simulink model "modelo_dp_mod_am"  (R2024b)
settings: Solver=VariableStepDiscrete  StartTime=0.0  StopTime=sim_time  RelTol=1e-3  EnableMultiTasking=on
values from neighbouring files (symbols this model uses):
  f_cic_scale = ceil(log2(G_cic_int))    [conf_mod_filter_design_p1_2.m]
  fc = 30    [configura_modelo_dp_mod_am.m]
  fmod = 20    [configura_modelo_dp_mod_am.m]
  fsc = 96    [configura_modelo_dp_mod_am.m]
  h_comp_cic = round(h_comp_cic*2^16)*2^-16    [conf_mod_filter_design_p1_2.m]
  h_comp_DAC = [-1/16 1-2^-3 -1/16]    [conf_mod_filter_design_p1_2.m]
  m_am = 1*(1-2^-15)    (= 0.999969482422)    [configura_modelo_dp_mod_am.m]
  R = 2000    [conf_mod_filter_design_p1_2.m]
undefined symbols (not defined in the file or in its folder): dspblkCoreblockFVToolHelper, gcbh
libraries: dspsigops x4, simulink x1, dspsrcs4 x1
settings Model: Creator=jvalls  LastModifiedBy=garto
settings SolverCC: AlgebraicLoopSolver=TrustRegion
settings DataIOCC: LimitDataPoints=on  SaveFormat=Array  ReturnWorkspaceOutputs=off
settings OptimizationCC: LifeSpan=inf
settings DebuggingCC: SolverPrmCheckMsg=warning  UnconnectedInputMsg=warning  UnconnectedOutputMsg=warning  UnconnectedLineMsg=warning  SFUnexpectedBacktrackingDiag=warning  SFNoUnconditionalDefaultTransitionDiag=warning  SFExecutionAtInitializationDiag=none  ArithmeticOperatorsInVariantConditions=warning
settings HardwareCC: ProdBitPerPointer=32  ProdBitPerSizeT=32  ProdBitPerPtrDiffT=32  ProdLargestAtomicFloat=None  ProdIntDivRoundTo=Undefined  ProdEndianess=Unspecified  ProdWordSize=32  ProdHWDeviceType=32-bit Generic
settings ModelReferenceCC: EnableRefExpFcnMdlSchedulingChecks=on  PropagateSignalLabelsOutOfModel=off
settings SFSimCC: SimUseLocalCustomCode=off  CustomCodeUndefinedFunction=UseInterfaceOnly
settings RTWCC: RTWUseLocalCustomCode=off  GPUComputeCapability=3.5
settings CodeAppCC: StateflowObjectComments=on
settings GRTTargetCC: TargetLangStandard=C89/C90 (ANSI)
settings ConfigComp: CovMetricSettings=dw  CovSaveCumulativeToWorkspaceVar=on  CovSaveSingleToWorkspaceVar=on  CovExternalEMLEnable=off  CovSFcnEnable=off

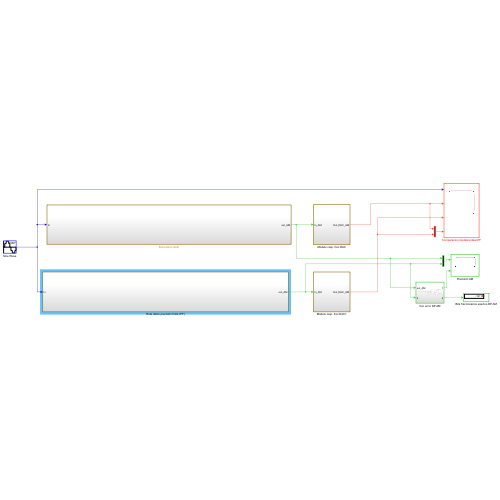
[thumbnail: Simulink's stored preview of the top-level diagram]
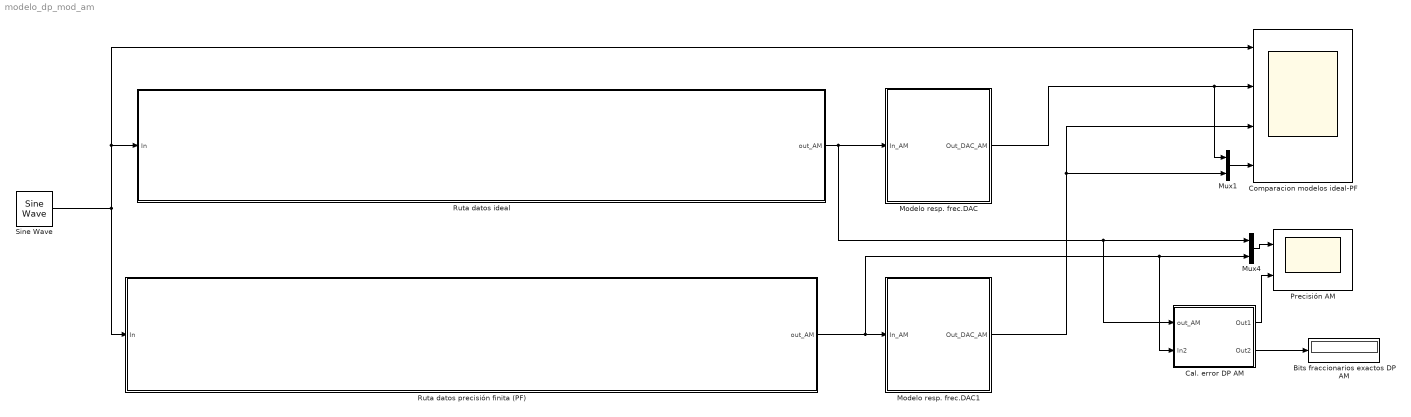
== system modelo_dp_mod_am ==
  Bits fraccionarios exactos DP AM : Display
  Cal. error DP AM : Subsystem
  Comparacion modelos ideal-PF : Scope  NumInputPorts=4
  Modelo resp. frec.DAC : Subsystem
  Modelo resp. frec.DAC1 : Subsystem
  Mux1 : Mux  Inputs=2
  Mux4 : Mux  Inputs=2
  Precisión AM : Scope  NumInputPorts=2
  Ruta datos ideal : Subsystem
  Ruta datos precisión finita (PF) : Subsystem
  Sine Wave : dspsrcs4/Sine Wave  Amplitude=1-2^-15  Frequency=fmod*1e-3  Phase=0  SampleMode=Discrete  OutComplex=Real  CompMethod=Trigonometric fcn  TableSize=Speed  SampleTime=R/fsc  SamplesPerFrame=1  ResetState=Restart at time zero  OutputFrames=off  dataType=double  wordLen=16  udDataType=sfix(16)  fracBitsMode=Best precision  numFracBits=15  OutDataTypeStr=double  LastOutDataTypeStr=double
  wires:
  Mux1/1 -> Comparacion modelos ideal-PF/4
  Modelo resp. frec.DAC/1(Out_DAC_AM) -> Mux1/1, Comparacion modelos ideal-PF/2
  Modelo resp. frec.DAC1/1(Out_DAC_AM) -> Comparacion modelos ideal-PF/3, Mux1/2
  Ruta datos ideal/1(out_AM) -> Cal. error DP AM/1(out_AM), Mux4/1, Modelo resp. frec.DAC/1(In_AM)
  Ruta datos precisión finita (PF)/1(out_AM) -> Cal. error DP AM/2(In2), Mux4/2, Modelo resp. frec.DAC1/1(In_AM)
  Cal. error DP AM/1(Out1) -> Precisión AM/2
  Cal. error DP AM/2(Out2) -> Bits fraccionarios exactos DP AM/1
  Sine Wave/1 -> Comparacion modelos ideal-PF/1, Ruta datos ideal/1(In), Ruta datos precisión finita (PF)/1(In)
  Mux4/1 -> Precisión AM/1

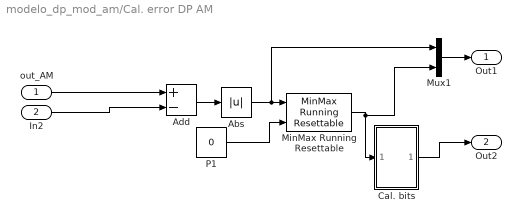
== system modelo_dp_mod_am/Cal. error DP AM ==
  out_AM : Inport
  In2 : Inport  Port=2
  Abs : Abs  SaturateOnIntegerOverflow=off
  Add : Sum  Inputs=+-
  Cal. bits : Subsystem
  MinMax Running Resettable : simulink/Math Operations/MinMax Running Resettable  Function=max  vinit=0.0
  Mux1 : Mux  Inputs=2
  P1 : Constant  Value=0  OutDataTypeStr=double  SampleTime=-1
  Out1 : Outport  VectorParamsAs1DForOutWhenUnconnected=off
  Out2 : Outport  Port=2  VectorParamsAs1DForOutWhenUnconnected=off
  wires:
  In2/1 -> Add/2
  Abs/1 -> Mux1/1, MinMax Running Resettable/1
  MinMax Running Resettable/1 -> Mux1/2, Cal. bits/1(In1)
  out_AM/1 -> Add/1
  P1/1 -> MinMax Running Resettable/2
  Add/1 -> Abs/1
  Cal. bits/1(Out1) -> Out2/1
  Mux1/1 -> Out1/1

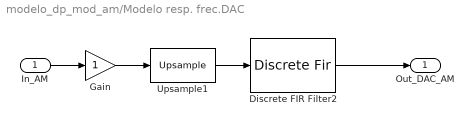
== system modelo_dp_mod_am/Modelo resp. frec.DAC ==
  In_AM : Inport
  Discrete FIR Filter2 : DiscreteFir  Coefficients=[1 1 1 1]  InputProcessing=Columns as channels (frame based)
  Gain : Gain  OutDataTypeStr=double
  Upsample1 : dspsigops/Upsample  FactorSource=Dialog parameter  N=4  Nmax=16  phase=0  InputProcessing=Columns as channels (frame based)  RateOptions=Allow multirate processing  ic=0  mode=Unused parameter value
  Out_DAC_AM : Outport  VectorParamsAs1DForOutWhenUnconnected=off
  wires:
  Upsample1/1 -> Discrete FIR Filter2/1
  Discrete FIR Filter2/1 -> Out_DAC_AM/1
  In_AM/1 -> Gain/1
  Gain/1 -> Upsample1/1

== system modelo_dp_mod_am/Modelo resp. frec.DAC1 ==
  In_AM : Inport
  Discrete FIR Filter2 : DiscreteFir  Coefficients=[1 1 1 1]  InputProcessing=Columns as channels (frame based)
  Gain : Gain  OutDataTypeStr=double
  Upsample1 : dspsigops/Upsample  FactorSource=Dialog parameter  N=4  Nmax=16  phase=0  InputProcessing=Columns as channels (frame based)  RateOptions=Allow multirate processing  ic=0  mode=Unused parameter value
  Out_DAC_AM : Outport  VectorParamsAs1DForOutWhenUnconnected=off
  wires:
  Upsample1/1 -> Discrete FIR Filter2/1
  Discrete FIR Filter2/1 -> Out_DAC_AM/1
  In_AM/1 -> Gain/1
  Gain/1 -> Upsample1/1

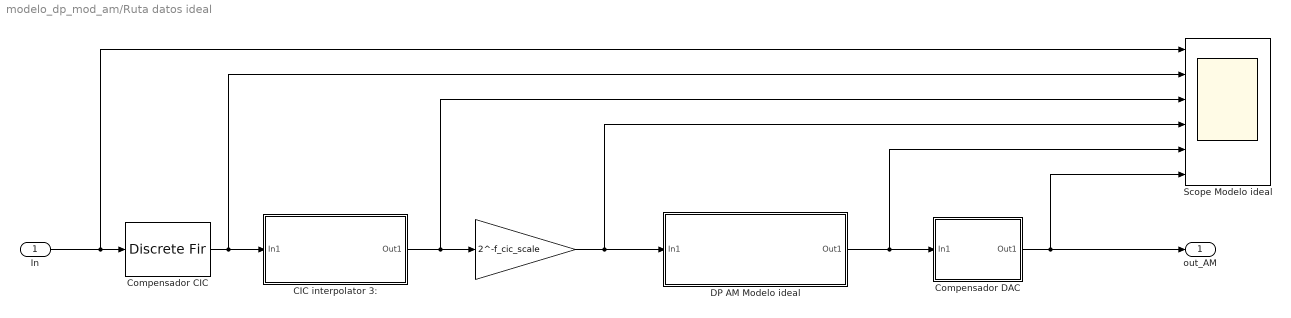
== system modelo_dp_mod_am/Ruta datos ideal ==
  In : Inport
  " " : Gain  Gain=2^-f_cic_scale  OutDataTypeStr=double
  "CIC interpolator 3: " : Subsystem
  Compensador CIC : DiscreteFir  LoadFcn=dspblkCoreblockFVToolHelper(gcbh,'load');  Coefficients=h_comp_cic  InputProcessing=Columns as channels (frame based)
      settings: CopyFcn=dspblkCoreblockFVToolHelper(gcbh,'copy');  DeleteFcn=dspblkCoreblockFVToolHelper(gcbh,'close');  ModelCloseFcn=dspblkCoreblockFVToolHelper(gcbh,'close');  PreSaveFcn=dspblkCoreblockFVToolHelper(gcbh,'presave');  PostSaveFcn=dspblkCoreblockFVToolHelper(gcbh,'postsave');  CloseFcn=dspblkCoreblockFVToolHelper(gcbh,'close');
  Compensador DAC : Subsystem
  DP AM Modelo ideal : Subsystem
  Scope Modelo ideal : Scope  NumInputPorts=6
  out_AM : Outport  VectorParamsAs1DForOutWhenUnconnected=off
  wires:
  "CIC interpolator 3: "/1(Out1) -> Scope Modelo ideal/3, " "/1
  " "/1 -> Scope Modelo ideal/4, DP AM Modelo ideal/1(In1)
  In/1 -> Scope Modelo ideal/1, Compensador CIC/1
  DP AM Modelo ideal/1(Out1) -> Compensador DAC/1(In1), Scope Modelo ideal/5
  Compensador CIC/1 -> Scope Modelo ideal/2, "CIC interpolator 3: "/1(In1)
  Compensador DAC/1(Out1) -> Scope Modelo ideal/6, out_AM/1

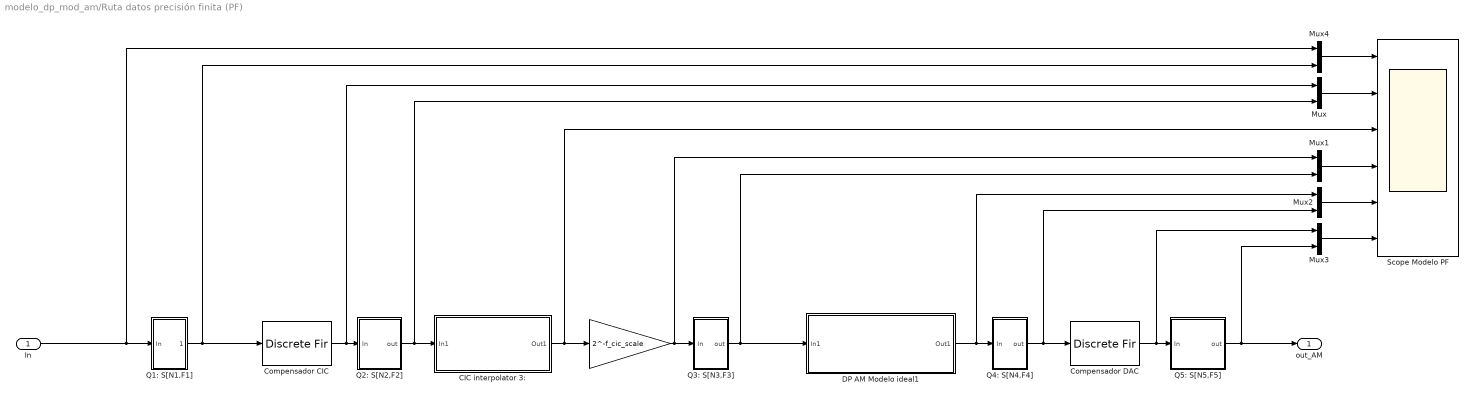
== system modelo_dp_mod_am/Ruta datos precisión finita (PF) ==
  In : Inport
  " " : Gain  Gain=2^-f_cic_scale  OutDataTypeStr=double
  "CIC interpolator 3: " : Subsystem
  Compensador CIC : DiscreteFir  LoadFcn=dspblkCoreblockFVToolHelper(gcbh,'load');  Coefficients=h_comp_cic  InputProcessing=Columns as channels (frame based)
      settings: CopyFcn=dspblkCoreblockFVToolHelper(gcbh,'copy');  DeleteFcn=dspblkCoreblockFVToolHelper(gcbh,'close');  ModelCloseFcn=dspblkCoreblockFVToolHelper(gcbh,'close');  PreSaveFcn=dspblkCoreblockFVToolHelper(gcbh,'presave');  PostSaveFcn=dspblkCoreblockFVToolHelper(gcbh,'postsave');  CloseFcn=dspblkCoreblockFVToolHelper(gcbh,'close');
  Compensador DAC : DiscreteFir  Coefficients=h_comp_DAC  InputProcessing=Columns as channels (frame based)
  DP AM Modelo ideal1 : Subsystem
  Mux{,1..4} (5 alike) : Mux  Inputs=2
  Q1: S[N1,F1] : Subsystem
  Q2: S[N2,F2] : Subsystem
  Q3: S[N3,F3] : Subsystem
  Q4: S[N4,F4] : Subsystem
  Q5: S[N5,F5] : Subsystem
  Scope Modelo PF : Scope  NumInputPorts=6
  out_AM : Outport  VectorParamsAs1DForOutWhenUnconnected=off
  wires:
  Compensador CIC/1 -> Mux/1, Q2: S[N2,F2]/1(In)
  " "/1 -> Q3: S[N3,F3]/1(In), Mux1/1
  DP AM Modelo ideal1/1(Out1) -> Mux2/1, Q4: S[N4,F4]/1(In)
  In/1 -> Mux4/1, Q1: S[N1,F1]/1(In)
  Q2: S[N2,F2]/1(out) -> Mux/2, "CIC interpolator 3: "/1(In1)
  Q3: S[N3,F3]/1(out) -> Mux1/2, DP AM Modelo ideal1/1(In1)
  Q5: S[N5,F5]/1(out) -> Mux3/2, out_AM/1
  "CIC interpolator 3: "/1(Out1) -> Scope Modelo PF/3, " "/1
  Q4: S[N4,F4]/1(out) -> Compensador DAC/1, Mux2/2
  Compensador DAC/1 -> Mux3/1, Q5: S[N5,F5]/1(In)
  Mux/1 -> Scope Modelo PF/2
  Mux1/1 -> Scope Modelo PF/4
  Mux2/1 -> Scope Modelo PF/5
  Mux3/1 -> Scope Modelo PF/6
  Q1: S[N1,F1]/1(Out1) -> Mux4/2, Compensador CIC/1
  Mux4/1 -> Scope Modelo PF/1

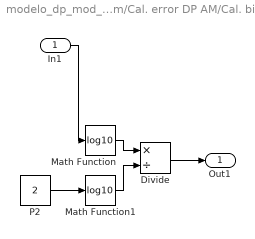
== system modelo_dp_mod_am/Cal. error DP AM/Cal. bits ==
  In1 : Inport
  Divide : Product  Inputs=*/
  Math Function : Math  Operator=log10  SignedPower=on
  Math Function1 : Math  Operator=log10  SignedPower=on
  P2 : Constant  Value=2  OutDataTypeStr=double  SampleTime=-1
  Out1 : Outport  VectorParamsAs1DForOutWhenUnconnected=off
  wires:
  P2/1 -> Math Function1/1
  Math Function1/1 -> Divide/2
  In1/1 -> Math Function/1
  Math Function/1 -> Divide/1
  Divide/1 -> Out1/1

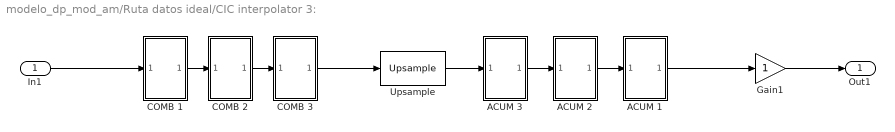
== system modelo_dp_mod_am/Ruta datos ideal/CIC interpolator 3:  ==
  In1 : Inport
  ACUM 1 : Subsystem
  ACUM 2 : Subsystem
  ACUM 3 : Subsystem
  COMB 1 : Subsystem
  COMB 2 : Subsystem
  COMB 3 : Subsystem
  Gain1 : Gain  OutDataTypeStr=double
  Upsample : dspsigops/Upsample  FactorSource=Dialog parameter  N=R  Nmax=16  phase=0  InputProcessing=Columns as channels (frame based)  RateOptions=Allow multirate processing  ic=0  mode=Unused parameter value
  Out1 : Outport  VectorParamsAs1DForOutWhenUnconnected=off
  wires:
  ACUM 1/1(Out1) -> Gain1/1
  In1/1 -> COMB 1/1(In1)
  COMB 1/1(Out1) -> COMB 2/1(In1)
  COMB 2/1(Out1) -> COMB 3/1(In1)
  ACUM 2/1(Out1) -> ACUM 1/1(In1)
  Upsample/1 -> ACUM 3/1(In1)
  ACUM 3/1(Out1) -> ACUM 2/1(In1)
  COMB 3/1(Out1) -> Upsample/1
  Gain1/1 -> Out1/1

== system modelo_dp_mod_am/Ruta datos ideal/Compensador DAC ==
  In1 : Inport
  Compensador DAC : DiscreteFir  Coefficients=h_comp_DAC  InputProcessing=Columns as channels (frame based)
  Multiply : Gain  OutDataTypeStr=double
  Out1 : Outport
  wires:
  Compensador DAC/1 -> Multiply/1
  In1/1 -> Compensador DAC/1
  Multiply/1 -> Out1/1

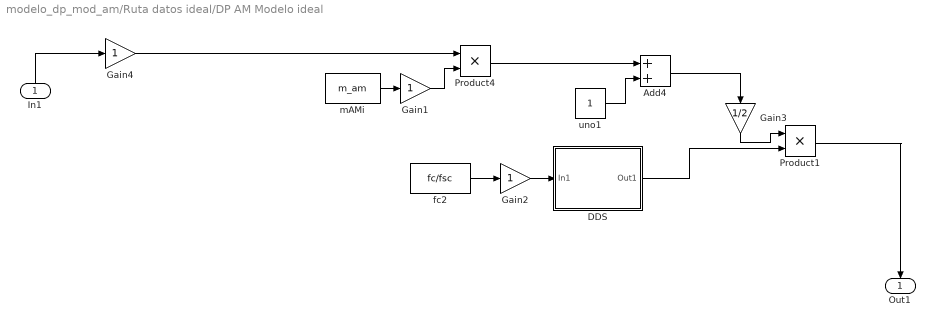
== system modelo_dp_mod_am/Ruta datos ideal/DP AM Modelo ideal ==
  In1 : Inport
  Add4 : Sum
  DDS : Subsystem
  Gain1 : Gain  OutDataTypeStr=double
  Gain2 : Gain  OutDataTypeStr=double
  Gain3 : Gain  Gain=1/2  OutDataTypeStr=double
  Gain4 : Gain  OutDataTypeStr=double
  Product1 : Product
  Product4 : Product
  fc2 : Constant  Value=fc/fsc  OutDataTypeStr=fixdt(0,24,24)
  "mAMi " : Constant  Value=m_am  OutDataTypeStr=fixdt(0,16,15)
  uno1 : Constant
  Out1 : Outport  VectorParamsAs1DForOutWhenUnconnected=off
  wires:
  Product1/1 -> Out1/1
  Gain3/1 -> Product1/1
  In1/1 -> Gain4/1
  Add4/1 -> Gain3/1
  uno1/1 -> Add4/2
  Product4/1 -> Add4/1
  "mAMi "/1 -> Gain1/1
  DDS/1(Out1) -> Product1/2
  fc2/1 -> Gain2/1
  Gain1/1 -> Product4/2
  Gain2/1 -> DDS/1(In1)
  Gain4/1 -> Product4/1

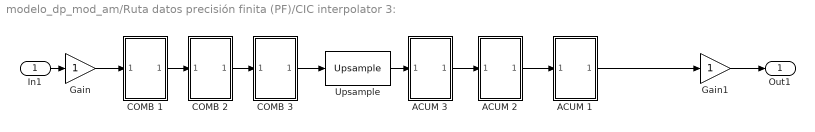
== system modelo_dp_mod_am/Ruta datos precisión finita (PF)/CIC interpolator 3:  ==
  In1 : Inport
  ACUM 1 : Subsystem
  ACUM 2 : Subsystem
  ACUM 3 : Subsystem
  COMB 1 : Subsystem
  COMB 2 : Subsystem
  COMB 3 : Subsystem
  Gain : Gain  OutDataTypeStr=double
  Gain1 : Gain  OutDataTypeStr=double
  Upsample : dspsigops/Upsample  FactorSource=Dialog parameter  N=R  Nmax=16  phase=0  InputProcessing=Columns as channels (frame based)  RateOptions=Allow multirate processing  ic=0  mode=Unused parameter value
  Out1 : Outport  VectorParamsAs1DForOutWhenUnconnected=off
  wires:
  ACUM 1/1(Out1) -> Gain1/1
  COMB 1/1(Out1) -> COMB 2/1(In1)
  COMB 2/1(Out1) -> COMB 3/1(In1)
  ACUM 2/1(Out1) -> ACUM 1/1(In1)
  Upsample/1 -> ACUM 3/1(In1)
  ACUM 3/1(Out1) -> ACUM 2/1(In1)
  COMB 3/1(Out1) -> Upsample/1
  Gain1/1 -> Out1/1
  In1/1 -> Gain/1
  Gain/1 -> COMB 1/1(In1)

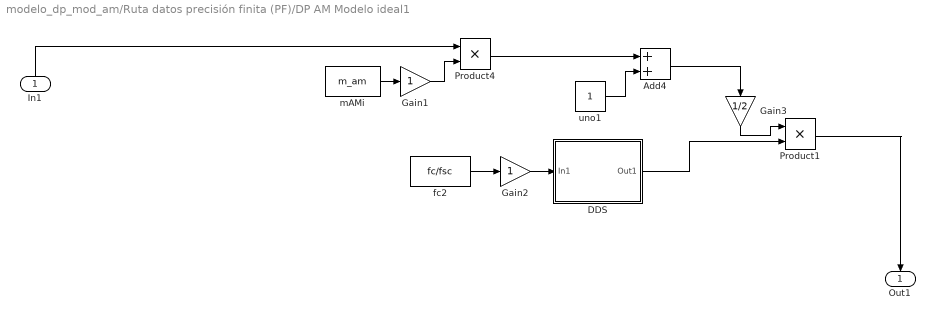
== system modelo_dp_mod_am/Ruta datos precisión finita (PF)/DP AM Modelo ideal1 ==
  In1 : Inport
  Add4 : Sum
  DDS : Subsystem
  Gain1 : Gain  OutDataTypeStr=double
  Gain2 : Gain  OutDataTypeStr=double
  Gain3 : Gain  Gain=1/2  OutDataTypeStr=double
  Product1 : Product
  Product4 : Product
  fc2 : Constant  Value=fc/fsc  OutDataTypeStr=fixdt(0,24,24)
  "mAMi " : Constant  Value=m_am  OutDataTypeStr=fixdt(0,16,15)
  uno1 : Constant
  Out1 : Outport  VectorParamsAs1DForOutWhenUnconnected=off
  wires:
  Product1/1 -> Out1/1
  Gain3/1 -> Product1/1
  Add4/1 -> Gain3/1
  uno1/1 -> Add4/2
  Product4/1 -> Add4/1
  "mAMi "/1 -> Gain1/1
  DDS/1(Out1) -> Product1/2
  fc2/1 -> Gain2/1
  Gain1/1 -> Product4/2
  Gain2/1 -> DDS/1(In1)
  In1/1 -> Product4/1

== system modelo_dp_mod_am/Ruta datos precisión finita (PF)/Q1: S[N1,F1] ==
  In : Inport
  Gain4 : Gain  OutDataTypeStr=double
  Q1: S[N1,F1]] : Gain  OutDataTypeStr=fixdt(1,N1,F1)
  Out1 : Outport  VectorParamsAs1DForOutWhenUnconnected=off
  wires:
  In/1 -> Q1: S[N1,F1]]/1
  Q1: S[N1,F1]]/1 -> Gain4/1
  Gain4/1 -> Out1/1

== system modelo_dp_mod_am/Ruta datos precisión finita (PF)/Q2: S[N2,F2] ==
  In : Inport
  Gain4 : Gain  OutDataTypeStr=double
  Q2: S[N2,F2] : Gain  OutDataTypeStr=fixdt(1,N2,F2)
  out : Outport  VectorParamsAs1DForOutWhenUnconnected=off
  wires:
  In/1 -> Q2: S[N2,F2]/1
  Q2: S[N2,F2]/1 -> Gain4/1
  Gain4/1 -> out/1

== system modelo_dp_mod_am/Ruta datos precisión finita (PF)/Q3: S[N3,F3] ==
  In : Inport
  Gain4 : Gain  OutDataTypeStr=double
  Q3: S[N3,F3] : Gain  OutDataTypeStr=fixdt(1,N3,F3)
  out : Outport  VectorParamsAs1DForOutWhenUnconnected=off
  wires:
  In/1 -> Q3: S[N3,F3]/1
  Q3: S[N3,F3]/1 -> Gain4/1
  Gain4/1 -> out/1

== system modelo_dp_mod_am/Ruta datos precisión finita (PF)/Q4: S[N4,F4] ==
  In : Inport
  Gain4 : Gain  OutDataTypeStr=double
  Q4: S[N4,F4] : Gain  OutDataTypeStr=fixdt(1,N4,F4)
  out : Outport  VectorParamsAs1DForOutWhenUnconnected=off
  wires:
  In/1 -> Q4: S[N4,F4]/1
  Q4: S[N4,F4]/1 -> Gain4/1
  Gain4/1 -> out/1

== system modelo_dp_mod_am/Ruta datos precisión finita (PF)/Q5: S[N5,F5] ==
  In : Inport
  Gain4 : Gain  OutDataTypeStr=double
  Q5: S[N5,F5] : Gain  OutDataTypeStr=fixdt(1,N5,F5)
  out : Outport  VectorParamsAs1DForOutWhenUnconnected=off
  wires:
  In/1 -> Q5: S[N5,F5]/1
  Q5: S[N5,F5]/1 -> Gain4/1
  Gain4/1 -> out/1

== system modelo_dp_mod_am/Ruta datos ideal/CIC interpolator 3: /ACUM 1 ==
  In1 : Inport
  "   Integer Delay " : Delay  DelayLength=1
  Add11 : Sum
  Out1 : Outport  VectorParamsAs1DForOutWhenUnconnected=off
  wires:
  In1/1 -> Add11/2
  Add11/1 -> Out1/1, "   Integer Delay "/1
  "   Integer Delay "/1 -> Add11/1

== system modelo_dp_mod_am/Ruta datos ideal/CIC interpolator 3: /ACUM 2 ==
  In1 : Inport
  "   Integer Delay " : Delay  DelayLength=1
  Add11 : Sum
  Out1 : Outport  VectorParamsAs1DForOutWhenUnconnected=off
  wires:
  In1/1 -> Add11/2
  Add11/1 -> Out1/1, "   Integer Delay "/1
  "   Integer Delay "/1 -> Add11/1

== system modelo_dp_mod_am/Ruta datos ideal/CIC interpolator 3: /ACUM 3 ==
  In1 : Inport
  "   Integer Delay " : Delay  DelayLength=1
  Add11 : Sum
  Out1 : Outport  VectorParamsAs1DForOutWhenUnconnected=off
  wires:
  In1/1 -> Add11/2
  Add11/1 -> Out1/1, "   Integer Delay "/1
  "   Integer Delay "/1 -> Add11/1

== system modelo_dp_mod_am/Ruta datos ideal/CIC interpolator 3: /COMB 1 ==
  In1 : Inport
  Add8 : Sum  Inputs=+-
  "Integer Delay " : Delay  DelayLength=1
  Out1 : Outport  VectorParamsAs1DForOutWhenUnconnected=off
  wires:
  Add8/1 -> Out1/1
  In1/1 -> "Integer Delay "/1, Add8/1
  "Integer Delay "/1 -> Add8/2

== system modelo_dp_mod_am/Ruta datos ideal/CIC interpolator 3: /COMB 2 ==
  In1 : Inport
  Add8 : Sum  Inputs=+-
  "Integer Delay " : Delay  DelayLength=1
  Out1 : Outport  VectorParamsAs1DForOutWhenUnconnected=off
  wires:
  Add8/1 -> Out1/1
  In1/1 -> "Integer Delay "/1, Add8/1
  "Integer Delay "/1 -> Add8/2

== system modelo_dp_mod_am/Ruta datos ideal/CIC interpolator 3: /COMB 3 ==
  In1 : Inport
  Add8 : Sum  Inputs=+-
  "Integer Delay " : Delay  DelayLength=1
  Out1 : Outport  VectorParamsAs1DForOutWhenUnconnected=off
  wires:
  Add8/1 -> Out1/1
  In1/1 -> "Integer Delay "/1, Add8/1
  "Integer Delay "/1 -> Add8/2

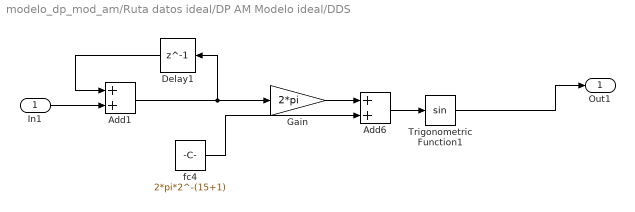
== system modelo_dp_mod_am/Ruta datos ideal/DP AM Modelo ideal/DDS ==
  In1 : Inport
  Add1 : Sum
  Add6 : Sum
  Delay1 : Delay  DelayLength=1
  Gain : Gain  Gain=2*pi
  Trigonometric Function1 : Trigonometry
  fc4 : Constant  Value=2*pi*2^-(15+1)
  Out1 : Outport  VectorParamsAs1DForOutWhenUnconnected=off
  wires:
  Trigonometric Function1/1 -> Out1/1
  Add6/1 -> Trigonometric Function1/1
  Add1/1 -> Delay1/1, Gain/1
  In1/1 -> Add1/2
  fc4/1 -> Add6/2
  Gain/1 -> Add6/1
  Delay1/1 -> Add1/1

== system modelo_dp_mod_am/Ruta datos precisión finita (PF)/CIC interpolator 3: /ACUM 1 ==
  In1 : Inport
  "   Integer Delay " : Delay  DelayLength=1
  Add11 : Sum
  Out1 : Outport  VectorParamsAs1DForOutWhenUnconnected=off
  wires:
  In1/1 -> Add11/2
  Add11/1 -> Out1/1, "   Integer Delay "/1
  "   Integer Delay "/1 -> Add11/1

== system modelo_dp_mod_am/Ruta datos precisión finita (PF)/CIC interpolator 3: /ACUM 2 ==
  In1 : Inport
  "   Integer Delay " : Delay  DelayLength=1
  Add11 : Sum
  Out1 : Outport  VectorParamsAs1DForOutWhenUnconnected=off
  wires:
  In1/1 -> Add11/2
  Add11/1 -> Out1/1, "   Integer Delay "/1
  "   Integer Delay "/1 -> Add11/1

== system modelo_dp_mod_am/Ruta datos precisión finita (PF)/CIC interpolator 3: /ACUM 3 ==
  In1 : Inport
  "   Integer Delay " : Delay  DelayLength=1
  Add11 : Sum
  Out1 : Outport  VectorParamsAs1DForOutWhenUnconnected=off
  wires:
  In1/1 -> Add11/2
  Add11/1 -> Out1/1, "   Integer Delay "/1
  "   Integer Delay "/1 -> Add11/1

== system modelo_dp_mod_am/Ruta datos precisión finita (PF)/CIC interpolator 3: /COMB 1 ==
  In1 : Inport
  Add8 : Sum  Inputs=+-
  "Integer Delay " : Delay  DelayLength=1
  Out1 : Outport  VectorParamsAs1DForOutWhenUnconnected=off
  wires:
  Add8/1 -> Out1/1
  In1/1 -> "Integer Delay "/1, Add8/1
  "Integer Delay "/1 -> Add8/2

== system modelo_dp_mod_am/Ruta datos precisión finita (PF)/CIC interpolator 3: /COMB 2 ==
  In1 : Inport
  Add8 : Sum  Inputs=+-
  "Integer Delay " : Delay  DelayLength=1
  Out1 : Outport  VectorParamsAs1DForOutWhenUnconnected=off
  wires:
  Add8/1 -> Out1/1
  In1/1 -> "Integer Delay "/1, Add8/1
  "Integer Delay "/1 -> Add8/2

== system modelo_dp_mod_am/Ruta datos precisión finita (PF)/CIC interpolator 3: /COMB 3 ==
  In1 : Inport
  Add8 : Sum  Inputs=+-
  "Integer Delay " : Delay  DelayLength=1
  Out1 : Outport  VectorParamsAs1DForOutWhenUnconnected=off
  wires:
  Add8/1 -> Out1/1
  In1/1 -> "Integer Delay "/1, Add8/1
  "Integer Delay "/1 -> Add8/2

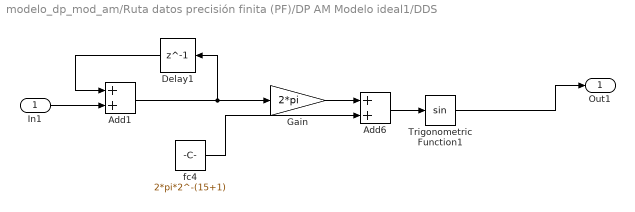
== system modelo_dp_mod_am/Ruta datos precisión finita (PF)/DP AM Modelo ideal1/DDS ==
  In1 : Inport
  Add1 : Sum
  Add6 : Sum
  Delay1 : Delay  DelayLength=1
  Gain : Gain  Gain=2*pi
  Trigonometric Function1 : Trigonometry
  fc4 : Constant  Value=2*pi*2^-(15+1)
  Out1 : Outport  VectorParamsAs1DForOutWhenUnconnected=off
  wires:
  Trigonometric Function1/1 -> Out1/1
  Add6/1 -> Trigonometric Function1/1
  Add1/1 -> Delay1/1, Gain/1
  In1/1 -> Add1/2
  fc4/1 -> Add6/2
  Gain/1 -> Add6/1
  Delay1/1 -> Add1/1
